simulink model "CE1"  (R2018a)
settings: Solver=VariableStepAuto  StartTime=0.0  StopTime=40  RelTol=1e-3
settings Model: Creator=linky  LastModifiedBy=linky

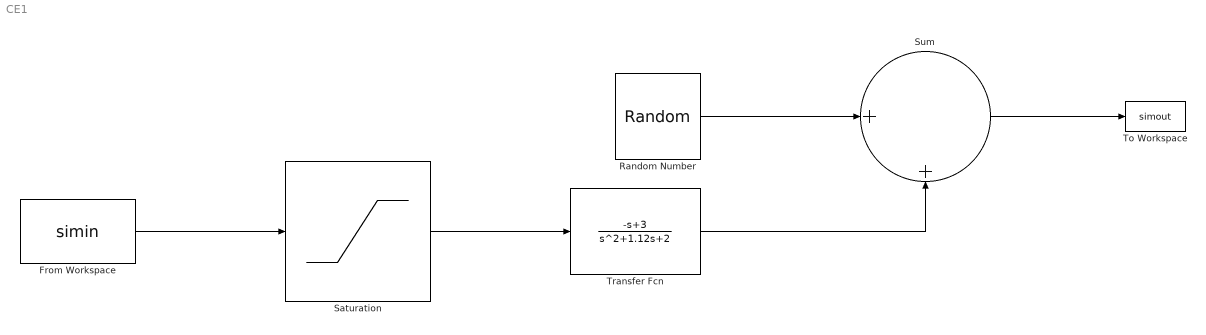
== system CE1 ==
  From Workspace : FromWorkspace  VariableName=simin  SampleTime=0.1
  Random Number : RandomNumber  Variance=0.02  SampleTime=0.1
  Saturation : Saturate
  Sum : Sum  Inputs=|++
  To Workspace : ToWorkspace  VariableName=simout  SaveFormat=Timeseries  SampleTime=0.1
  Transfer Fcn : TransferFcn  Numerator=[-1 3]  Denominator=[1 1.12 2]
  wires:
  Transfer Fcn/1 -> Sum/2
  From Workspace/1 -> Saturation/1
  Saturation/1 -> Transfer Fcn/1
  Sum/1 -> To Workspace/1
  Random Number/1 -> Sum/1
